simulink model "Simulink_Schuurmans"  (Simulink 8.2)
settings: Solver=ode4  SolverMode=SingleTasking  StartTime=0.0  StopTime=300  FixedStep=0.01  RelTol=1e-3
InitFcn:
  | Main;
values from neighbouring files (symbols this model uses):
  A1 = [   1   0.1 ... (first row only)    [Matrizes.m]    (also in MatrizesEspacoEstados.m)
  B1 = [0 ... (first row only)    [Matrizes.m]    (also in MatrizesEspacoEstados.m)
  C = eye(n)    [Matrizes.m]    (also in MatrizesEspacoEstados.m)
  D = 0*C(:,n)    [Matrizes.m]    (also in MatrizesEspacoEstados.m)
undefined symbols (not defined in the file or in its folder): xk0
undefined symbols (not defined in the file): A, B, Umax
settings Model: Creator=Kawakami  LastModifiedBy=Eduardo
settings DataIOCC: LimitDataPoints=off  SaveOutput=off  SaveTime=off  TimeSaveName=t  SignalLoggingName=sigsOut
settings OptimizationCC: BooleanDataType=off
settings DebuggingCC: SaveWithParameterizedLinksMsg=none  SignalResolutionControl=TryResolveAllWithWarning  SolverPrmCheckMsg=none  MultiTaskDSMMsg=warning  MultiTaskCondExecSysMsg=none
settings HardwareCC: TargetUnknown=on
settings RTWCC: IncludeERTFirstTime=on

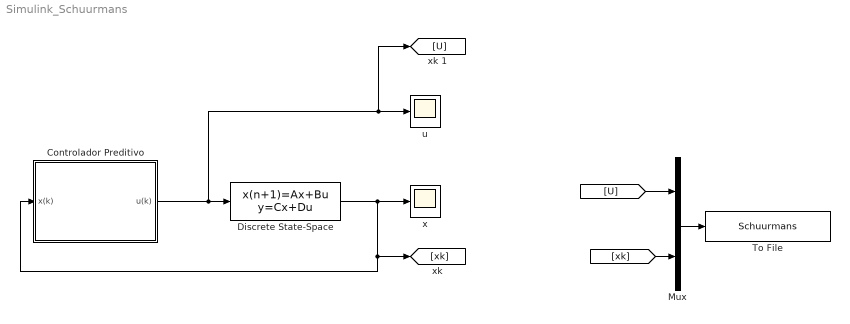
== system Simulink_Schuurmans ==
  "Controlador Preditivo  " : Subsystem  mask{A=A, B=B, Umax=Umax, T=1}
      mask prompts: A "Matriz Agregada A"; B "Matriz Agregada B"; T "T (passo da simulação)"
  Discrete State-Space : DiscreteStateSpace  A=A1  B=B1  C=C  D=D  X0=xk0
  Mux : Mux  Inputs=2
  To File : ToFile  Filename=Schuurmans  MatrixName=Schuurmans
  u : Scope
      settings: TimeRange=10  YMin=0.000175  YMax=0.0005
  x : Scope
      settings: YMin=-1.25  YMax=2.25
  wires:
  "Controlador Preditivo  "/1(u(k)) -> [U], u/1, Discrete State-Space/1
  Discrete State-Space/1 -> x/1, [xk], "Controlador Preditivo  "/1(x(k))
  Mux/1 -> To File/1
  [xk] -> Mux/2
  [U] -> Mux/1

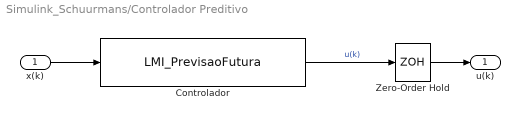
== system Simulink_Schuurmans/Controlador Preditivo   ==
  x(k) : Inport
  Controlador : S-Function  FunctionName=LMI_PrevisaoFutura  Parameters=A, B, Umax, T  EnableBusSupport=off
  Zero-Order Hold : ZeroOrderHold  SampleTime=T
  u(k) : Outport
  wires:
  Zero-Order Hold/1 -> u(k)/1
  x(k)/1 -> Controlador/1
  Controlador/1 -> Zero-Order Hold/1  "u(k)"
